simulink model "DockingLTI_Model"  (R2024b)
settings: Solver=VariableStepAuto  StartTime=0.0  StopTime=inf  RelTol=1e-3
undefined symbols (not defined in the file or in its folder): sat
libraries: cstblocks x1
settings Model: Creator=Ameya  LastModifiedBy=Ameya

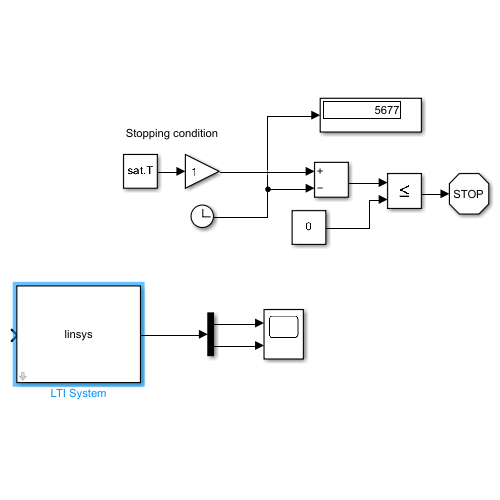
[thumbnail: Simulink's stored preview of the top-level diagram]
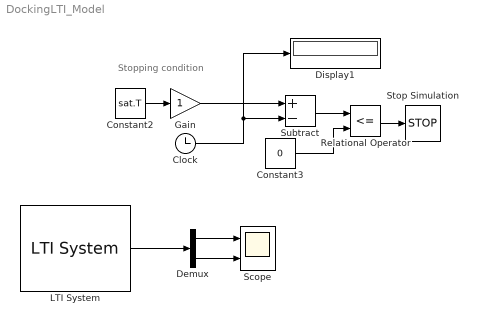
== system DockingLTI_Model ==
  note: Stopping condition
  Clock : Clock
  Constant2 : Constant  Value=sat.T
  Constant3 : Constant  Value=0
  Demux : Demux  Outputs=2
  Display1 : Display
  Gain : Gain
  LTI System : cstblocks/LTI System  sys=linsys  IC=[0;0;1;0;0;0.15]  PadeOrder=0
  Relational Operator : RelationalOperator  Operator=<=  OutDataTypeStr=boolean  RndMeth=Simplest  InputSameDT=off
  Scope : Scope  NumInputPorts=2
  Stop Simulation : Stop
  Subtract : Sum  Inputs=+-
  wires:
  LTI System/1 -> Demux/1
  Demux/1 -> Scope/1
  Demux/2 -> Scope/2
  Relational Operator/1 -> Stop Simulation/1
  Clock/1 -> Display1/1, Subtract/2
  Gain/1 -> Subtract/1
  Subtract/1 -> Relational Operator/1
  Constant2/1 -> Gain/1
  Constant3/1 -> Relational Operator/2
